simulink model "rx2"  (R2022b)
settings: Solver=FixedStepDiscrete  StartTime=0.0  StopTime=3.3E6  FixedStep=1  RelTol=1e-3  EnableMultiTasking=on
model workspace (MAT data in the model file):
  mwTaskManagerKernelLatency = 0
undefined symbols (not defined in the file or in its folder): Add, jsin, magnitude, rom_pilot_conj_tt, Shift
libraries: hdlsllib x3231, whdlutilities x525, simulink x260, whdlmod x112, whdledac x26, dsphdlmathfun2 x24, commchan3 x1
(part 8 of 59)

== system rx2/process11/decoder/p-p ==
  data_in : Inport  OutDataTypeStr=boolean  PortDimensions=64
  start_in : Inport  Port=2  OutDataTypeStr=boolean  PortDimensions=1
  valid : Inport  Port=3  OutDataTypeStr=boolean  PortDimensions=1
  Compare To Constant : hdlsllib/Logic and Bit Operations/Compare To Constant  relop===  const=64  OutDataTypeStr=boolean
  Compare To Constant1 : hdlsllib/Logic and Bit Operations/Compare To Constant  relop=<=  const=72  OutDataTypeStr=boolean
  Compare To Constant2 : hdlsllib/Logic and Bit Operations/Compare To Constant  relop===  const=1  OutDataTypeStr=boolean
  Compare To Constant3 : hdlsllib/Logic and Bit Operations/Compare To Constant  relop===  const=528  OutDataTypeStr=boolean
  Compare To Constant4 : hdlsllib/Logic and Bit Operations/Compare To Constant  relop=<=  const=528  OutDataTypeStr=boolean
  Delay : Delay  DelayLength=1  InitialCondition=0
  Delay1 : Delay  DelayLength=1  InitialCondition=0
  Ground : Ground
  HDL Counter : hdlsllib/Sources/HDL Counter  CountType=Count limited  CountInit=0  CountStep=1  CountMax=2000  CountFromType=Specify  CountFrom=0  CountResetPort=on  CountLoadPort=off  CountEnbPort=on  CountDirPort=off  CountHitOutputPort=off  CountDataType=Unsigned  CountWordLen=16  CountFracLen=0  CountSampTime=1
  HDL Counter1 : hdlsllib/Sources/HDL Counter  CountType=Count limited  CountInit=1  CountStep=1  CountMax=64  CountFromType=Specify  CountFrom=1  CountResetPort=on  CountLoadPort=off  CountEnbPort=on  CountDirPort=off  CountHitOutputPort=off  CountDataType=Unsigned  CountWordLen=16  CountFracLen=0  CountSampTime=1
  HDL Counter2 : hdlsllib/Sources/HDL Counter  CountType=Count limited  CountInit=0  CountStep=1  CountMax=100  CountFromType=Specify  CountFrom=0  CountResetPort=on  CountLoadPort=off  CountEnbPort=on  CountDirPort=off  CountHitOutputPort=off  CountDataType=Unsigned  CountWordLen=16  CountFracLen=0  CountSampTime=1
  HDL Counter3 : hdlsllib/Sources/HDL Counter  CountType=Count limited  CountInit=1  CountStep=1  CountMax=64*2  CountFromType=Initial value  CountFrom=1  CountResetPort=on  CountLoadPort=off  CountEnbPort=on  CountDirPort=off  CountHitOutputPort=off  CountDataType=Unsigned  CountWordLen=8  CountFracLen=0  CountSampTime=1
  HDL Counter4 : hdlsllib/Sources/HDL Counter  CountType=Count limited  CountInit=0  CountStep=1  CountMax=1000  CountFromType=Initial value  CountFrom=0  CountResetPort=on  CountLoadPort=off  CountEnbPort=on  CountDirPort=off  CountHitOutputPort=off  CountDataType=Unsigned  CountWordLen=16  CountFracLen=0  CountSampTime=1
  HDL Counter5 : hdlsllib/Sources/HDL Counter  CountType=Count limited  CountInit=1  CountStep=1  CountMax=1000  CountFromType=Initial value  CountFrom=1  CountResetPort=on  CountLoadPort=off  CountEnbPort=on  CountDirPort=off  CountHitOutputPort=off  CountDataType=Unsigned  CountWordLen=16  CountFracLen=0  CountSampTime=1
  Logical Operator1 : Logic  Operator=NOT  AllPortsSameDT=off  OutDataTypeStr=boolean
  Logical Operator2 : Logic  Operator=NOT  AllPortsSameDT=off  OutDataTypeStr=boolean
  Logical Operator3 : Logic  AllPortsSameDT=off  OutDataTypeStr=boolean
  Logical Operator5 : Logic  Operator=NOT  AllPortsSameDT=off  OutDataTypeStr=boolean
  Logical Operator6 : Logic  AllPortsSameDT=off  OutDataTypeStr=boolean
  Sample Control Bus Creator : whdlutilities/Sample Control Bus Creator
  Subsystem : Subsystem  mask{valid_length=20*64}
      mask prompts: valid_length "The length of valid"
      mask DialogControl Control2 Prompt: Latency=2
  Subsystem2 : Subsystem  mask{data_type=boolean, address_len=16}
      mask prompts: data_type "the type of input data"; address_len "the length of address"
      mask DialogControl ParameterGroupVar Prompt: 参数
  Switch : Switch  Criteria=u2 ~= 0  SaturateOnIntegerOverflow=off  InputSameDT=off
  p_s_new : Subsystem
  data : Outport
  ctrl : Outport  Port=2
  wires:
  Ground/1 -> Switch/3
  Switch/1 -> data/1
  Subsystem/3(end_out) -> p_s_new/3(end)
  p_s_new/1(data_out) -> Delay1/1
  Subsystem2/1(rd_dout) -> p_s_new/1(data_in)
  Subsystem/1(valid_out) -> HDL Counter1/2, Logical Operator1/1, HDL Counter3/2, Logical Operator2/1, Logical Operator3/1, p_s_new/2(valid)
  Logical Operator6/1 -> HDL Counter4/2, Delay/1
  Compare To Constant4/1 -> Logical Operator6/1
  HDL Counter5/1 -> Compare To Constant4/1
  Sample Control Bus Creator/1 -> ctrl/1
  Delay1/1 -> Switch/1
  Delay/1 -> Sample Control Bus Creator/3, Switch/2
  Compare To Constant3/1 -> HDL Counter4/1, Sample Control Bus Creator/2
  Compare To Constant2/1 -> Sample Control Bus Creator/1
  HDL Counter1/1 -> Compare To Constant/1
  Compare To Constant1/1 -> Logical Operator3/2
  HDL Counter3/1 -> Compare To Constant1/1
  HDL Counter2/1 -> Subsystem2/4(rd_addr)
  data_in/1 -> Subsystem2/1(data1)
  Logical Operator5/1 -> HDL Counter/1
  Logical Operator2/1 -> HDL Counter3/1, HDL Counter5/1
  Compare To Constant/1 -> HDL Counter2/2
  start_in/1 -> Subsystem/1(start)
  HDL Counter/1 -> Subsystem2/2(wr_addr)
  valid/1 -> Logical Operator5/1, Subsystem2/3(wr_en1), HDL Counter/2
  Logical Operator3/1 -> Logical Operator6/2, HDL Counter5/2
  Logical Operator1/1 -> HDL Counter1/1, HDL Counter2/1
  HDL Counter4/1 -> Compare To Constant2/1, Compare To Constant3/1

== system rx2/process11/decoder/rate recover ==
  demod : Inport
  valid_in : Inport  Port=2
  start_in : Inport  Port=3
  Compare To Constant : hdlsllib/Logic and Bit Operations/Compare To Constant  relop=<=  const=384  OutDataTypeStr=boolean
  Compare To Constant1 : hdlsllib/Logic and Bit Operations/Compare To Constant  relop=>=  const=577  OutDataTypeStr=boolean
  Compare To Constant2 : hdlsllib/Logic and Bit Operations/Compare To Constant  relop=<=  const=1776  OutDataTypeStr=boolean
  Compare To Constant3 : hdlsllib/Logic and Bit Operations/Compare To Constant  relop=>=  const=385  OutDataTypeStr=boolean
  Compare To Constant4 : hdlsllib/Logic and Bit Operations/Compare To Constant  relop=<=  const=576  OutDataTypeStr=boolean
  Compare To Constant5 : hdlsllib/Logic and Bit Operations/Compare To Constant  relop=>=  const=1777  OutDataTypeStr=boolean
  Compare To Constant6 : hdlsllib/Logic and Bit Operations/Compare To Constant  relop=<=  const=3600  OutDataTypeStr=boolean
  Constant : Constant  Value=0
  Constant1 : Constant  Value=0
  Delay{,1..4} (5 alike) : Delay  InitialCondition=0
  HDL Counter : hdlsllib/Sources/HDL Counter  CountType=Count limited  CountInit=1  CountStep=1  CountMax=10000  CountFromType=Initial value  CountFrom=1  CountResetPort=on  CountLoadPort=off  CountEnbPort=on  CountDirPort=off  CountHitOutputPort=off  CountDataType=Unsigned  CountWordLen=16  CountFracLen=0  CountSampTime=1
  HDL Counter1 : hdlsllib/Sources/HDL Counter  CountType=Count limited  CountInit=0  CountStep=1  CountMax=10000  CountFromType=Initial value  CountFrom=0  CountResetPort=on  CountLoadPort=off  CountEnbPort=on  CountDirPort=off  CountHitOutputPort=off  CountDataType=Unsigned  CountWordLen=16  CountFracLen=0  CountSampTime=1
  HDL Counter3 : hdlsllib/Sources/HDL Counter  CountType=Count limited  CountInit=1  CountStep=1  CountMax=10000  CountFromType=Initial value  CountFrom=1  CountResetPort=on  CountLoadPort=off  CountEnbPort=on  CountDirPort=off  CountHitOutputPort=off  CountDataType=Unsigned  CountWordLen=16  CountFracLen=0  CountSampTime=1
  Logical Operator : Logic  Operator=NOT  AllPortsSameDT=off  OutDataTypeStr=boolean
  Logical Operator{1,3..4,6..7} (5 alike) : Logic  AllPortsSameDT=off  OutDataTypeStr=boolean
  Logical Operator5 : Logic  Operator=OR  AllPortsSameDT=off  OutDataTypeStr=boolean
  Logical Operator8 : Logic  Operator=NOT  AllPortsSameDT=off  OutDataTypeStr=boolean
  Simple Dual Port RAM : hdlsllib/HDL RAMs/Simple Dual Port RAM  ram_size=16
  Subsystem : Subsystem  mask{valid_length=3600}
      mask prompts: valid_length "The length of valid"
      mask DialogControl Control2 Prompt: Latency=2
  Switch : Switch  Criteria=u2 ~= 0  SaturateOnIntegerOverflow=off  InputSameDT=off
  Switch1 : Switch  Criteria=u2 ~= 0  OutDataTypeStr=fixdt(1,16,9)  SaturateOnIntegerOverflow=off  InputSameDT=off
  rate_recover : Outport  PortDimensions=1
  start_out : Outport  Port=2  OutDataTypeStr=boolean
  end_out : Outport  Port=3  OutDataTypeStr=boolean
  valid_out : Outport  Port=4  OutDataTypeStr=boolean
  wires:
  Compare To Constant5/1 -> Logical Operator4/1
  Logical Operator3/1 -> Delay3/1
  Subsystem/1(valid_out) -> Logical Operator8/1, Logical Operator6/2, Delay/1, HDL Counter3/2
  Constant1/1 -> Switch1/1
  Subsystem/2(start_out) -> Delay1/1  "start"
  Logical Operator/1 -> HDL Counter/1
  Logical Operator1/1 -> Logical Operator5/2
  Compare To Constant3/1 -> Logical Operator3/1
  Subsystem/3(end_out) -> Delay2/1  "end"
  HDL Counter/1 -> Simple Dual Port RAM/2  "wr_addr"
  Compare To Constant6/1 -> Logical Operator4/2
  Compare To Constant1/1 -> Logical Operator1/1
  Compare To Constant2/1 -> Logical Operator1/2
  valid_in/1 -> Simple Dual Port RAM/3, HDL Counter/2, Logical Operator/1
  Delay1/1 -> start_out/1  "start_out"
  Logical Operator7/1 -> Delay4/1  "3"
  Simple Dual Port RAM/1 -> Switch/3  "rd_dout"
  start_in/1 -> Subsystem/1(start)
  Compare To Constant4/1 -> Logical Operator3/2
  Logical Operator4/1 -> Logical Operator7/1
  Constant/1 -> Switch/1
  Switch/1 -> Switch1/3  "2_out"
  Switch1/1 -> rate_recover/1  "data_out"
  Logical Operator5/1 -> Logical Operator6/1
  Compare To Constant/1 -> Logical Operator5/1
  Delay2/1 -> end_out/1  "end_out"
  demod/1 -> Simple Dual Port RAM/1
  Delay/1 -> Logical Operator7/2, valid_out/1  "valid_out"
  Logical Operator8/1 -> HDL Counter1/1, HDL Counter3/1
  HDL Counter3/1 -> Compare To Constant1/1, Compare To Constant/1, Compare To Constant6/1, Compare To Constant5/1, Compare To Constant4/1, Compare To Constant3/1, Compare To Constant2/1  "count"
  Delay3/1 -> Switch/2  "2"
  Delay4/1 -> Switch1/2  "3"
  Logical Operator6/1 -> HDL Counter1/2  "1"
  HDL Counter1/1 -> Simple Dual Port RAM/4  "rd_addr"

== system rx2/process11/decoder/s-p ==
  data_in : Inport
  valid_in : Inport  Port=2
  Compare To Constant1 : hdlsllib/Logic and Bit Operations/Compare To Constant  relop=<=  const=64  OutDataTypeStr=boolean
  Compare To Constant2 : hdlsllib/Logic and Bit Operations/Compare To Constant  relop===  const=2  OutDataTypeStr=boolean
  Compare To Constant3 : hdlsllib/Logic and Bit Operations/Compare To Constant  relop===  const=3  OutDataTypeStr=boolean
  Compare To Constant4 : hdlsllib/Logic and Bit Operations/Compare To Constant  relop===  const=1  OutDataTypeStr=boolean
  Compare To Constant5 : hdlsllib/Logic and Bit Operations/Compare To Constant  relop===  const=100  OutDataTypeStr=boolean
  Constant2 : Constant  Value=2  OutDataTypeStr=uint8
  Constant3 : Constant  Value=zeros(1,56)  OutDataTypeStr=fixdt(1,16,9)
  Delay1 : Delay  DelayLength=1  InitialCondition=0
  Delay4 : Delay  DelayLength=1  InitialCondition=0
  HDL Counter : hdlsllib/Sources/HDL Counter  CountType=Count limited  CountInit=1  CountStep=1  CountMax=72  CountFromType=Initial value  CountFrom=1  CountResetPort=on  CountLoadPort=off  CountEnbPort=on  CountDirPort=off  CountHitOutputPort=off  CountDataType=Unsigned  CountWordLen=8  CountFracLen=0  CountSampTime=1
  HDL Counter1 : hdlsllib/Sources/HDL Counter  CountType=Count limited  CountInit=1  CountStep=1  CountMax=72  CountFromType=Initial value  CountFrom=1  CountResetPort=on  CountLoadPort=off  CountEnbPort=on  CountDirPort=off  CountHitOutputPort=off  CountDataType=Unsigned  CountWordLen=8  CountFracLen=0  CountSampTime=1
  HDL Counter2 : hdlsllib/Sources/HDL Counter  CountType=Count limited  CountInit=1  CountStep=1  CountMax=72  CountFromType=Initial value  CountFrom=1  CountResetPort=on  CountLoadPort=off  CountEnbPort=on  CountDirPort=off  CountHitOutputPort=off  CountDataType=Unsigned  CountWordLen=8  CountFracLen=0  CountSampTime=1
  HDL Counter3 : hdlsllib/Sources/HDL Counter  CountType=Count limited  CountInit=0  CountStep=1  CountMax=200  CountFromType=Initial value  CountFrom=0  CountResetPort=on  CountLoadPort=off  CountEnbPort=on  CountDirPort=off  CountHitOutputPort=off  CountDataType=Unsigned  CountWordLen=8  CountFracLen=0  CountSampTime=1
  Logical Operator{1,5..6,8} (4 alike) : Logic  Operator=NOT  AllPortsSameDT=off  OutDataTypeStr=boolean
  Logical Operator2 : Logic  Operator=XOR  AllPortsSameDT=off  OutDataTypeStr=boolean
  Logical Operator3 : Logic  AllPortsSameDT=off  OutDataTypeStr=boolean
  Logical Operator4 : Logic  AllPortsSameDT=off  OutDataTypeStr=boolean
  Mod : Math  Operator=mod
  Mux : Mux  Inputs=2
  S-P : Subsystem  mask{data_len=64}
      mask prompts: data_len "the length of parallel"
      mask DialogControl ParameterGroupVar Prompt: 参数
  S-P2 : Subsystem  mask{data_len=8}
      mask prompts: data_len "the length of parallel"
      mask DialogControl ParameterGroupVar Prompt: 参数
  Sample Control Bus Creator : whdlutilities/Sample Control Bus Creator
  Switch1 : Switch  Criteria=u2 ~= 0  OutDataTypeStr=Inherit: Inherit via back propagation  SaturateOnIntegerOverflow=off  InputSameDT=off
  data_out : Outport
  ctrl_out : Outport  Port=2
  wires:
  Compare To Constant1/1 -> Logical Operator8/1, Logical Operator3/2
  Logical Operator2/1 -> Delay1/1, HDL Counter3/2  "valid"
  Logical Operator4/1 -> Sample Control Bus Creator/1  "start"
  HDL Counter/1 -> Compare To Constant1/1
  Compare To Constant2/1 -> Logical Operator2/1, Delay4/1
  S-P2/2(valid_out) -> HDL Counter2/2, Logical Operator6/1
  HDL Counter1/1 -> Compare To Constant2/1
  data_in/1 -> S-P2/1(data_in), S-P/1(data_in)
  valid_in/1 -> Logical Operator1/1, Logical Operator3/1, HDL Counter/2
  Sample Control Bus Creator/1 -> ctrl_out/1
  Constant3/1 -> Mux/2
  HDL Counter3/1 -> Mod/1, Compare To Constant4/1, Compare To Constant5/1
  Compare To Constant3/1 -> Logical Operator2/2
  Mod/1 -> Switch1/2
  Switch1/1 -> data_out/1
  Constant2/1 -> Mod/2
  S-P2/1(data_out) -> Mux/1
  Mux/1 -> Switch1/3
  HDL Counter2/1 -> Compare To Constant3/1
  Logical Operator8/1 -> S-P2/2(valid_in)
  S-P/2(valid_out) -> HDL Counter1/2, Logical Operator5/1  "validout"
  S-P/1(data_out) -> Switch1/1
  Logical Operator3/1 -> S-P/2(valid_in)
  Logical Operator1/1 -> HDL Counter/1
  Logical Operator5/1 -> HDL Counter1/1
  Logical Operator6/1 -> HDL Counter2/1
  Compare To Constant5/1 -> Sample Control Bus Creator/2, HDL Counter3/1  "start"
  Compare To Constant4/1 -> Logical Operator4/2
  Delay4/1 -> Logical Operator4/1
  Delay1/1 -> Sample Control Bus Creator/3

== system rx2/process11/decoder/soft demodule ==
  nVar_tt : Inport  OutDataTypeStr=fixdt(0,16,12)
  G_k_1 : Inport  Port=2
  r_k : Inport  Port=3
  start : Inport  Port=4
  valid : Inport  Port=5
  Complex to Real-Imag : ComplexToRealImag
  Constant1 : Constant  Value=2  OutDataTypeStr=uint16
  Constant2 : Constant  Value=2  OutDataTypeStr=uint16
  Constant3 : Constant  Value=0  OutDataTypeStr=uint16
  Constant4 : Constant  Value=0  OutDataTypeStr=uint16
  Data Type Conversion2 : DataTypeConversion  OutDataTypeStr=boolean  SaturateOnIntegerOverflow=off  RndMeth=Floor
  Delay1 : Delay  InitialCondition=0
  Delay2 : Delay  DelayLength=1  InitialCondition=0
  Delay3 : Delay  InitialCondition=0
  Delay4 : Delay  InitialCondition=0
  HDL Counter : hdlsllib/Sources/HDL Counter  CountType=Count limited  CountInit=1  CountStep=1  CountMax=2000  CountFromType=Initial value  CountFrom=1  CountResetPort=on  CountLoadPort=off  CountEnbPort=on  CountDirPort=off  CountHitOutputPort=off  CountDataType=Unsigned  CountWordLen=16  CountFracLen=0  CountSampTime=1
  HDL Counter2 : hdlsllib/Sources/HDL Counter  CountType=Count limited  CountInit=1  CountStep=1  CountMax=2000  CountFromType=Initial value  CountFrom=1  CountResetPort=on  CountLoadPort=off  CountEnbPort=on  CountDirPort=off  CountHitOutputPort=off  CountDataType=Unsigned  CountWordLen=16  CountFracLen=0  CountSampTime=1
  HDL Counter3 : hdlsllib/Sources/HDL Counter  CountType=Count limited  CountInit=0  CountStep=1  CountMax=2000  CountFromType=Initial value  CountFrom=0  CountResetPort=on  CountLoadPort=off  CountEnbPort=on  CountDirPort=off  CountHitOutputPort=off  CountDataType=Unsigned  CountWordLen=16  CountFracLen=0  CountSampTime=1
  HDL Counter5 : hdlsllib/Sources/HDL Counter  CountType=Count limited  CountInit=0  CountStep=1  CountMax=2000  CountFromType=Initial value  CountFrom=0  CountResetPort=on  CountLoadPort=off  CountEnbPort=on  CountDirPort=off  CountHitOutputPort=off  CountDataType=Unsigned  CountWordLen=16  CountFracLen=0  CountSampTime=1
  Logical Operator2 : Logic  AllPortsSameDT=off  OutDataTypeStr=boolean
  Logical Operator3 : Logic  Operator=NOT  AllPortsSameDT=off  OutDataTypeStr=boolean
  Logical Operator4 : Logic  Operator=NOT  AllPortsSameDT=off  OutDataTypeStr=boolean
  Logical Operator5 : Logic  Operator=NOT  AllPortsSameDT=off  OutDataTypeStr=boolean
  Logical Operator6 : Logic  Operator=XOR  AllPortsSameDT=off  OutDataTypeStr=boolean
  Math Reciprocal2 : Math  Operator=reciprocal  SignedPower=on  OutDataTypeStr=fixdt(1,16,12)
  Mod : Math  Operator=mod  SignedPower=on
  Product : Product
  Product1 : Product
  Product10 : Product  OutDataTypeStr=fixdt(1,35,24)
  Product2 : Product  OutDataTypeStr=fixdt(1,35,24)
  Simple Dual Port RAM : hdlsllib/HDL RAMs/Simple Dual Port RAM  ram_size=16
  Simple Dual Port RAM1 : hdlsllib/HDL RAMs/Simple Dual Port RAM  ram_size=16
  Subsystem : Subsystem  mask{valid_length=demod_length}
      mask prompts: valid_length "The length of valid"
      mask DialogControl Control2 Prompt: Latency=2
  Switch : Switch  Criteria=u2 ~= 0  SaturateOnIntegerOverflow=off  InputSameDT=off
  Switch1 : Switch  Criteria=u2 ~= 0  SaturateOnIntegerOverflow=off  InputSameDT=off
  Switch2 : Switch  Criteria=u2 ~= 0  SaturateOnIntegerOverflow=off  InputSameDT=off
  demod : Outport  OutDataTypeStr=fixdt(1,16,9)  VectorParamsAs1DForOutWhenUnconnected=off
  valid_out : Outport  Port=2  OutDataTypeStr=boolean  VectorParamsAs1DForOutWhenUnconnected=off
  start_out : Outport  Port=3  OutDataTypeStr=boolean  VectorParamsAs1DForOutWhenUnconnected=off
  end_out : Outport  Port=4  OutDataTypeStr=boolean  VectorParamsAs1DForOutWhenUnconnected=off
  wires:
  valid/1 -> Switch2/2, Switch1/2, Simple Dual Port RAM1/3, Simple Dual Port RAM/3, HDL Counter2/2, Logical Operator4/1  "valid_tt"
  start/1 -> Subsystem/1(start)
  Logical Operator2/1 -> Logical Operator6/2, HDL Counter3/2  "mod_1"
  Complex to Real-Imag/2 -> Product1/2  "r_k_imag"
  Subsystem/1(valid_out) -> Delay1/1, HDL Counter/2, Logical Operator3/1, Logical Operator2/2, Logical Operator6/1, Logical Operator5/1
  Product/1 -> Switch1/1  "demod_1"
  Product1/1 -> Switch2/1  "demod_0"
  Switch/1 -> demod/1  "demod"
  Mod/1 -> Data Type Conversion2/1  "mod"
  Logical Operator6/1 -> Delay2/1, HDL Counter5/2  "mod_0"
  Complex to Real-Imag/1 -> Product/2  "r_k_real"
  Logical Operator4/1 -> HDL Counter2/1
  HDL Counter3/1 -> Simple Dual Port RAM/4  "rd_addr1"
  Logical Operator5/1 -> HDL Counter5/1, HDL Counter3/1  "rst"
  Logical Operator3/1 -> HDL Counter/1
  Constant1/1 -> Mod/2
  HDL Counter5/1 -> Simple Dual Port RAM1/4  "rd_addr0"
  Simple Dual Port RAM/1 -> Switch/1  "demod_11"
  HDL Counter2/1 -> Simple Dual Port RAM1/2, Simple Dual Port RAM/2  "wr_addr"
  Simple Dual Port RAM1/1 -> Switch/3  "demod_00"
  Data Type Conversion2/1 -> Logical Operator2/1
  Delay1/1 -> valid_out/1  "valid_out"
  HDL Counter/1 -> Mod/1  "count"
  nVar_tt/1 -> Math Reciprocal2/1  "nvar"
  G_k_1/1 -> Product10/2  "G_k_1"
  r_k/1 -> Complex to Real-Imag/1  "r_k"
  Subsystem/2(start_out) -> Delay3/1
  Subsystem/3(end_out) -> Delay4/1
  Delay2/1 -> Switch/2
  Delay3/1 -> start_out/1  "start_out"
  Delay4/1 -> end_out/1  "end_out"
  Math Reciprocal2/1 -> Product10/1  "nvar"
  Product10/1 -> Product2/2
  Product2/1 -> Product1/1, Product/1
  Constant2/1 -> Product2/1
  Constant3/1 -> Switch1/3
  Switch1/1 -> Simple Dual Port RAM/1  "demod1"
  Constant4/1 -> Switch2/3
  Switch2/1 -> Simple Dual Port RAM1/1  "demod0"

== system rx2/process11/decoder/synchronization ==
  chan_est_tt : Inport
  rxSig_tt : Inport  Port=2
  port1_ctrl : Inport  Port=3  OutDataTypeStr=Bus: BUSOFDM1
  port2_ctrl : Inport  Port=4  OutDataTypeStr=Bus: BUSOFDM1
  Bus Selector1 : BusSelector  OutputSignals=signal1,signal2,signal3,signal4,signal5,signal6,signal7,signal8
  Bus Selector2 : BusSelector  OutputSignals=OFDM_ctrl_bf1_process1,OFDM_ctrl_bf1_process2,OFDM_ctrl_bf1_process3,OFDM_ctrl_bf1_process4,OFDM_ctrl_bf1_process5,OFDM_ctrl_bf1_process6,OFDM_ctrl_bf1_process7,OFDM_ctrl_bf1_process8
  Demux : Demux  Outputs=8
  Demux1 : Demux  Outputs=8
  Mux : Mux  Inputs=8
  Mux1 : Mux  Inputs=8
  data_synchronization1 : Subsystem
  data_synchronization2 : Subsystem
  data_synchronization3 : Subsystem
  data_synchronization4 : Subsystem
  data_synchronization5 : Subsystem
  data_synchronization6 : Subsystem
  data_synchronization7 : Subsystem
  data_synchronization8 : Subsystem
  port1_syn : Outport
  port2_syn : Outport  Port=2
  valid_syn : Outport  Port=3
  wires:
  Bus Selector2/3 -> data_synchronization8/4(port2_ctrl)  "<OFDM_ctrl_bf1_process3>"
  Bus Selector2/4 -> data_synchronization7/4(port2_ctrl)  "<OFDM_ctrl_bf1_process4>"
  Bus Selector2/5 -> data_synchronization6/4(port2_ctrl)  "<OFDM_ctrl_bf1_process5>"
  Bus Selector2/6 -> data_synchronization5/4(port2_ctrl)  "<OFDM_ctrl_bf1_process6>"
  Bus Selector2/7 -> data_synchronization4/4(port2_ctrl)  "<OFDM_ctrl_bf1_process7>"
  Bus Selector2/8 -> data_synchronization3/4(port2_ctrl)  "<OFDM_ctrl_bf1_process8>"
  Bus Selector2/2 -> data_synchronization2/4(port2_ctrl)  "<OFDM_ctrl_bf1_process2>"
  Bus Selector2/1 -> data_synchronization1/4(port2_ctrl)  "<OFDM_ctrl_bf1_process1>"
  port2_ctrl/1 -> Bus Selector2/1
  Bus Selector1/8 -> data_synchronization8/3(port1_ctrl)  "<signal8>"
  Bus Selector1/7 -> data_synchronization7/3(port1_ctrl)  "<signal7>"
  Bus Selector1/6 -> data_synchronization6/3(port1_ctrl)  "<signal6>"
  Bus Selector1/5 -> data_synchronization5/3(port1_ctrl)  "<signal5>"
  Bus Selector1/4 -> data_synchronization4/3(port1_ctrl)  "<signal4>"
  Bus Selector1/3 -> data_synchronization3/3(port1_ctrl)  "<signal3>"
  Bus Selector1/2 -> data_synchronization2/3(port1_ctrl)  "<signal2>"
  Bus Selector1/1 -> data_synchronization1/3(port1_ctrl)  "<signal1>"
  port1_ctrl/1 -> Bus Selector1/1
  rxSig_tt/1 -> Demux1/1
  data_synchronization6/3(valid_syn) -> ?
  chan_est_tt/1 -> Demux/1
  data_synchronization4/4(start_syn) -> ?
  data_synchronization2/3(valid_syn) -> ?
  data_synchronization4/3(valid_syn) -> ?
  data_synchronization6/4(start_syn) -> ?
  data_synchronization7/3(valid_syn) -> ?
  data_synchronization3/3(valid_syn) -> ?
  data_synchronization5/3(valid_syn) -> ?
  data_synchronization8/4(start_syn) -> ?
  Demux1/5 -> data_synchronization5/2(port2)
  Demux1/3 -> data_synchronization3/2(port2)
  data_synchronization2/4(start_syn) -> ?
  data_synchronization3/2(port2_syn) -> Mux1/3
  data_synchronization7/1(port1_syn) -> Mux/7
  Demux1/1 -> data_synchronization1/2(port2)
  Demux/8 -> data_synchronization8/1(port1)
  data_synchronization1/1(port1_syn) -> Mux/1
  Demux/3 -> data_synchronization3/1(port1)
  data_synchronization3/4(start_syn) -> ?
  data_synchronization1/3(valid_syn) -> valid_syn/1
  data_synchronization1/2(port2_syn) -> Mux1/1
  Demux/4 -> data_synchronization4/1(port1)
  data_synchronization5/4(start_syn) -> ?
  data_synchronization8/1(port1_syn) -> Mux/8
  Demux/6 -> data_synchronization6/1(port1)
  data_synchronization7/2(port2_syn) -> Mux1/7
  data_synchronization6/1(port1_syn) -> Mux/6
  Demux/7 -> data_synchronization7/1(port1)
  Demux/1 -> data_synchronization1/1(port1)
  data_synchronization4/2(port2_syn) -> Mux1/4
  data_synchronization4/1(port1_syn) -> Mux/4
  data_synchronization5/2(port2_syn) -> Mux1/5
  data_synchronization5/1(port1_syn) -> Mux/5
  Mux1/1 -> port2_syn/1
  Demux1/4 -> data_synchronization4/2(port2)
  Demux1/6 -> data_synchronization6/2(port2)
  data_synchronization8/2(port2_syn) -> Mux1/8
  data_synchronization2/2(port2_syn) -> Mux1/2
  data_synchronization7/4(start_syn) -> ?
  data_synchronization6/2(port2_syn) -> Mux1/6
  Demux/5 -> data_synchronization5/1(port1)
  Demux1/8 -> data_synchronization8/2(port2)
  data_synchronization8/3(valid_syn) -> ?
  Demux1/7 -> data_synchronization7/2(port2)
  data_synchronization2/1(port1_syn) -> Mux/2
  Mux/1 -> port1_syn/1
  Demux1/2 -> data_synchronization2/2(port2)
  Demux/2 -> data_synchronization2/1(port1)
  data_synchronization3/1(port1_syn) -> Mux/3

== system rx2/process11/decoder/synchronize_valid ==
  start : Inport
  Compare To Constant : simulink/Logic and Bit Operations/Compare To Constant  relop===  const=valid_length  OutDataTypeStr=boolean
  Data Type Conversion : DataTypeConversion  OutDataTypeStr=boolean  SaturateOnIntegerOverflow=off  RndMeth=Floor
  Delay2 : Delay  DelayLength=1  InitialCondition=0
  HDL Counter1 : hdlsllib/Sources/HDL Counter  CountType=Count limited  CountInit=1  CountStep=1  CountMax=valid_length  CountFromType=Initial value  CountFrom=1  CountResetPort=off  CountLoadPort=off  CountEnbPort=on  CountDirPort=off  CountHitOutputPort=off  CountDataType=Unsigned  CountWordLen=16  CountFracLen=0  CountSampTime=1
  HDL Counter4 : hdlsllib/Sources/HDL Counter  CountType=Count limited  CountInit=0  CountStep=1  CountMax=1  CountFromType=Initial value  CountFrom=0  CountResetPort=on  CountLoadPort=off  CountEnbPort=on  CountDirPort=off  CountHitOutputPort=off  CountDataType=Unsigned  CountWordLen=8  CountFracLen=0  CountSampTime=1
  valid_out : Outport
  wires:
  Compare To Constant/1 -> HDL Counter4/1
  HDL Counter1/1 -> Compare To Constant/1  "count_1"
  HDL Counter4/1 -> Data Type Conversion/1
  start/1 -> HDL Counter4/2
  Data Type Conversion/1 -> Delay2/1, HDL Counter1/1
  Delay2/1 -> valid_out/1  "valid_out"

== system rx2/process12/OFDM_DEMOD1/OFDM_demod1 ==
  ofdm_sym : Inport
  valid_in : Inport  Port=2  OutDataTypeStr=boolean
  OFDM Demodulator : whdlmod/OFDM Demodulator  OFDMParamsSource=Property  MaxFFTLength=64  FFTLength=1024  CPLength=72  NumLGsC=0  NumRGsC=0  CPFraction=off  CPFractionValue=0.55  removeDCSubcarriers=off  enableResetInputPort=off  Normalize=off  RoundingMethod=Floor  SimulateUsing=Code generation
  ctrl_gen : Subsystem
  data_out : Outport  OutDataTypeStr=fixdt(1,16,12)
  ctrl_out : Outport  Port=2  OutDataTypeStr=Bus: samplecontrol
  wires:
  ofdm_sym/1 -> OFDM Demodulator/1
  valid_in/1 -> OFDM Demodulator/2
  OFDM Demodulator/1 -> ctrl_gen/1(data_in)
  ctrl_gen/1(data_out) -> data_out/1
  OFDM Demodulator/2 -> ctrl_gen/2(valid_in)
  ctrl_gen/2(ctrl_out) -> ctrl_out/1

== system rx2/process12/OFDM_DEMOD1/OFDM_demod2 ==
  ofdm_sym : Inport
  valid_in : Inport  Port=2  OutDataTypeStr=boolean
  OFDM Demodulator : whdlmod/OFDM Demodulator  OFDMParamsSource=Property  MaxFFTLength=64  FFTLength=1024  CPLength=72  NumLGsC=0  NumRGsC=0  CPFraction=off  CPFractionValue=0.55  removeDCSubcarriers=off  enableResetInputPort=off  Normalize=off  RoundingMethod=Floor  SimulateUsing=Code generation
  ctrl_gen : Subsystem
  data_out : Outport  OutDataTypeStr=fixdt(1,16,12)
  ctrl_out : Outport  Port=2  OutDataTypeStr=Bus: samplecontrol
  wires:
  ofdm_sym/1 -> OFDM Demodulator/1
  valid_in/1 -> OFDM Demodulator/2
  OFDM Demodulator/1 -> ctrl_gen/1(data_in)
  ctrl_gen/1(data_out) -> data_out/1
  OFDM Demodulator/2 -> ctrl_gen/2(valid_in)
  ctrl_gen/2(ctrl_out) -> ctrl_out/1

== system rx2/process12/OFDM_DEMOD1/OFDM_demod3 ==
  ofdm_sym : Inport
  valid_in : Inport  Port=2  OutDataTypeStr=boolean
  OFDM Demodulator : whdlmod/OFDM Demodulator  OFDMParamsSource=Property  MaxFFTLength=64  FFTLength=1024  CPLength=72  NumLGsC=0  NumRGsC=0  CPFraction=off  CPFractionValue=0.55  removeDCSubcarriers=off  enableResetInputPort=off  Normalize=off  RoundingMethod=Floor  SimulateUsing=Code generation
  ctrl_gen : Subsystem
  data_out : Outport  OutDataTypeStr=fixdt(1,16,12)
  ctrl_out : Outport  Port=2  OutDataTypeStr=Bus: samplecontrol
  wires:
  ofdm_sym/1 -> OFDM Demodulator/1
  valid_in/1 -> OFDM Demodulator/2
  OFDM Demodulator/1 -> ctrl_gen/1(data_in)
  ctrl_gen/1(data_out) -> data_out/1
  OFDM Demodulator/2 -> ctrl_gen/2(valid_in)
  ctrl_gen/2(ctrl_out) -> ctrl_out/1

== system rx2/process12/OFDM_DEMOD1/OFDM_demod4 ==
  ofdm_sym : Inport
  valid_in : Inport  Port=2  OutDataTypeStr=boolean
  OFDM Demodulator : whdlmod/OFDM Demodulator  OFDMParamsSource=Property  MaxFFTLength=64  FFTLength=1024  CPLength=72  NumLGsC=0  NumRGsC=0  CPFraction=off  CPFractionValue=0.55  removeDCSubcarriers=off  enableResetInputPort=off  Normalize=off  RoundingMethod=Floor  SimulateUsing=Code generation
  ctrl_gen : Subsystem
  data_out : Outport  OutDataTypeStr=fixdt(1,16,12)
  ctrl_out : Outport  Port=2  OutDataTypeStr=Bus: samplecontrol
  wires:
  ofdm_sym/1 -> OFDM Demodulator/1
  valid_in/1 -> OFDM Demodulator/2
  OFDM Demodulator/1 -> ctrl_gen/1(data_in)
  ctrl_gen/1(data_out) -> data_out/1
  OFDM Demodulator/2 -> ctrl_gen/2(valid_in)
  ctrl_gen/2(ctrl_out) -> ctrl_out/1

== system rx2/process12/OFDM_DEMOD1/OFDM_demod5 ==
  ofdm_sym : Inport
  valid_in : Inport  Port=2  OutDataTypeStr=boolean
  OFDM Demodulator : whdlmod/OFDM Demodulator  OFDMParamsSource=Property  MaxFFTLength=64  FFTLength=1024  CPLength=72  NumLGsC=0  NumRGsC=0  CPFraction=off  CPFractionValue=0.55  removeDCSubcarriers=off  enableResetInputPort=off  Normalize=off  RoundingMethod=Floor  SimulateUsing=Code generation
  ctrl_gen : Subsystem
  data_out : Outport  OutDataTypeStr=fixdt(1,16,12)
  ctrl_out : Outport  Port=2  OutDataTypeStr=Bus: samplecontrol
  wires:
  ofdm_sym/1 -> OFDM Demodulator/1
  valid_in/1 -> OFDM Demodulator/2
  OFDM Demodulator/1 -> ctrl_gen/1(data_in)
  ctrl_gen/1(data_out) -> data_out/1
  OFDM Demodulator/2 -> ctrl_gen/2(valid_in)
  ctrl_gen/2(ctrl_out) -> ctrl_out/1

== system rx2/process12/OFDM_DEMOD1/OFDM_demod6 ==
  ofdm_sym : Inport
  valid_in : Inport  Port=2  OutDataTypeStr=boolean
  OFDM Demodulator : whdlmod/OFDM Demodulator  OFDMParamsSource=Property  MaxFFTLength=64  FFTLength=1024  CPLength=72  NumLGsC=0  NumRGsC=0  CPFraction=off  CPFractionValue=0.55  removeDCSubcarriers=off  enableResetInputPort=off  Normalize=off  RoundingMethod=Floor  SimulateUsing=Code generation
  ctrl_gen : Subsystem
  data_out : Outport  OutDataTypeStr=fixdt(1,16,12)
  ctrl_out : Outport  Port=2  OutDataTypeStr=Bus: samplecontrol
  wires:
  ofdm_sym/1 -> OFDM Demodulator/1
  valid_in/1 -> OFDM Demodulator/2
  OFDM Demodulator/1 -> ctrl_gen/1(data_in)
  ctrl_gen/1(data_out) -> data_out/1
  OFDM Demodulator/2 -> ctrl_gen/2(valid_in)
  ctrl_gen/2(ctrl_out) -> ctrl_out/1

== system rx2/process12/OFDM_DEMOD1/OFDM_demod7 ==
  ofdm_sym : Inport
  valid_in : Inport  Port=2  OutDataTypeStr=boolean
  OFDM Demodulator : whdlmod/OFDM Demodulator  OFDMParamsSource=Property  MaxFFTLength=64  FFTLength=1024  CPLength=72  NumLGsC=0  NumRGsC=0  CPFraction=off  CPFractionValue=0.55  removeDCSubcarriers=off  enableResetInputPort=off  Normalize=off  RoundingMethod=Floor  SimulateUsing=Code generation
  ctrl_gen : Subsystem
  data_out : Outport  OutDataTypeStr=fixdt(1,16,12)
  ctrl_out : Outport  Port=2  OutDataTypeStr=Bus: samplecontrol
  wires:
  ofdm_sym/1 -> OFDM Demodulator/1
  valid_in/1 -> OFDM Demodulator/2
  OFDM Demodulator/1 -> ctrl_gen/1(data_in)
  ctrl_gen/1(data_out) -> data_out/1
  OFDM Demodulator/2 -> ctrl_gen/2(valid_in)
  ctrl_gen/2(ctrl_out) -> ctrl_out/1

== system rx2/process12/OFDM_DEMOD1/OFDM_demod8 ==
  ofdm_sym : Inport
  valid_in : Inport  Port=2  OutDataTypeStr=boolean
  OFDM Demodulator : whdlmod/OFDM Demodulator  OFDMParamsSource=Property  MaxFFTLength=64  FFTLength=1024  CPLength=72  NumLGsC=0  NumRGsC=0  CPFraction=off  CPFractionValue=0.55  removeDCSubcarriers=off  enableResetInputPort=off  Normalize=off  RoundingMethod=Floor  SimulateUsing=Code generation
  ctrl_gen : Subsystem
  data_out : Outport  OutDataTypeStr=fixdt(1,16,12)
  ctrl_out : Outport  Port=2  OutDataTypeStr=Bus: samplecontrol
  wires:
  ofdm_sym/1 -> OFDM Demodulator/1
  valid_in/1 -> OFDM Demodulator/2
  OFDM Demodulator/1 -> ctrl_gen/1(data_in)
  ctrl_gen/1(data_out) -> data_out/1
  OFDM Demodulator/2 -> ctrl_gen/2(valid_in)
  ctrl_gen/2(ctrl_out) -> ctrl_out/1

== system rx2/process12/decoder/MRC ==
  chan_est_tt : Inport  OutDataTypeStr=fixdt(1,16,12)
  rxSig_tt : Inport  Port=2  OutDataTypeStr=fixdt(1,16,12)
  valid_tt : Inport  Port=3  OutDataTypeStr=boolean
  Add : Sum  Inputs=++++++++
  Add1 : Sum  Inputs=++++++++  OutDataTypeStr=fixdt(1,16,10)  SaturateOnIntegerOverflow=on
  Add2 : Sum  Inputs=++++++++  AccumDataTypeStr=fixdt(1,35,24)
  Constant : Constant  Value=0
  Constant1 : Constant  Value=0
  Demux : Demux  Outputs=8
  Demux1 : Demux  Outputs=8
  Detect Rise Positive1 : hdlsllib/Logic and Bit Operations/Detect Rise Positive  vinit=0  OutDataTypeStr=boolean
  Math Reciprocal : Math  Operator=reciprocal  SignedPower=on  OutDataTypeStr=fixdt(1,19,12)
  Math Reciprocal1 : Math  Operator=reciprocal  SignedPower=on
  Product : Product  OutDataTypeStr=fixdt(1,16,12)
  Product{1..8} (8 alike) : Product  OutDataTypeStr=fixdt(1,33,24)
  Product9 : Product  OutDataTypeStr=fixdt(1,16,9)
  Sqrt{1..8} (8 alike) : Sqrt  OutDataTypeStr=fixdt(1,16,12)  IntermediateResultsDataTypeStr=Inherit: Inherit from input
  Square{,1..7} (8 alike) : Math  Operator=magnitude^2  SignedPower=on  OutDataTypeStr=fixdt(1,32,24)  RndMeth=Zero
  Switch1 : Switch  Criteria=u2 ~= 0  SaturateOnIntegerOverflow=off  InputSameDT=off
  Switch2 : Switch  Criteria=u2 ~= 0  SaturateOnIntegerOverflow=off  InputSameDT=off
  Transpose{,1..7} (8 alike) : Math  Operator=hermitian  SignedPower=on  RndMeth=Zero
  G_k_1 : Outport
  r_k : Outport  Port=2
  start : Outport  Port=3  OutDataTypeStr=boolean  VectorParamsAs1DForOutWhenUnconnected=off
  valid : Outport  Port=4  OutDataTypeStr=boolean  VectorParamsAs1DForOutWhenUnconnected=off
  wires:
  Detect Rise Positive1/1 -> start/1
  Switch2/1 -> Product/1
  Constant1/1 -> Switch2/3
  Math Reciprocal/1 -> Switch2/1
  Constant/1 -> Switch1/3
  Switch1/1 -> Product9/1
  Math Reciprocal1/1 -> Switch1/1
  Product/1 -> G_k_1/1  "G_k_1"
  Demux1/2 -> Product2/2
  Square6/1 -> Add/7, Sqrt7/1
  Demux1/5 -> Product5/2
  Sqrt2/1 -> Add1/2
  Demux/5 -> Transpose4/1, Square4/1
  Sqrt5/1 -> Add1/5
  Product6/1 -> Add2/6
  Demux/1 -> Square/1, Transpose/1
  Sqrt1/1 -> Add1/1
  Product5/1 -> Add2/5
  Demux/3 -> Transpose2/1, Square2/1
  Transpose1/1 -> Product2/1
  Sqrt7/1 -> Add1/7
  Transpose2/1 -> Product3/1
  Demux1/3 -> Product3/2
  Square/1 -> Add/1, Sqrt1/1
  Demux1/1 -> Product1/2
  Transpose6/1 -> Product7/1
  Product9/1 -> r_k/1  "r_k"
  Product1/1 -> Add2/1
  Demux/6 -> Transpose5/1, Square5/1
  Add1/1 -> Math Reciprocal/1
  Product7/1 -> Add2/7
  Transpose5/1 -> Product6/1
  Transpose3/1 -> Product4/1
  Square3/1 -> Add/4, Sqrt4/1
  Sqrt3/1 -> Add1/3
  Product2/1 -> Add2/2
  valid_tt/1 -> valid/1, Switch2/2, Switch1/2, Detect Rise Positive1/1
  Square1/1 -> Add/2, Sqrt2/1
  Transpose4/1 -> Product5/1
  Product4/1 -> Add2/4
  Add/1 -> Product/2, Math Reciprocal1/1  "G_k"
  Demux/4 -> Transpose3/1, Square3/1
  rxSig_tt/1 -> Demux1/1
  Transpose/1 -> Product1/1
  Product3/1 -> Add2/3
  Transpose7/1 -> Product8/1
  Add2/1 -> Product9/2
  Square5/1 -> Add/6, Sqrt6/1
  Sqrt6/1 -> Add1/6
  chan_est_tt/1 -> Demux/1
  Demux1/6 -> Product6/2
  Demux1/8 -> Product8/2
  Square7/1 -> Add/8, Sqrt8/1
  Sqrt4/1 -> Add1/4
  Demux/7 -> Transpose6/1, Square6/1
  Sqrt8/1 -> Add1/8
  Demux1/4 -> Product4/2
  Product8/1 -> Add2/8
  Square4/1 -> Add/5, Sqrt5/1
  Square2/1 -> Add/3, Sqrt3/1
  Demux/2 -> Transpose1/1, Square1/1
  Demux1/7 -> Product7/2
  Demux/8 -> Transpose7/1, Square7/1

== system rx2/process12/decoder/deinterleave ==
  data_tt : Inport  SampleTime=1
  valid_tt : Inport  Port=2  OutDataTypeStr=boolean  SampleTime=1
  Compare To Constant : simulink/Logic and Bit Operations/Compare To Constant  relop=>  const=length/2-1  OutDataTypeStr=boolean
  Data Type Conversion : DataTypeConversion  OutDataTypeStr=boolean  SaturateOnIntegerOverflow=off  RndMeth=Floor
  Delay : Delay  DelayLength=1  InitialCondition=0
  Delay1 : Delay  DelayLength=1  InitialCondition=0
  Delay2 : Delay  DelayLength=1  InitialCondition=0
  Detect Fall Nonpositive : simulink/Logic and Bit Operations/Detect Fall Nonpositive  vinit=0  OutDataTypeStr=boolean
  Detect Rise Positive : simulink/Logic and Bit Operations/Detect Rise Positive  vinit=0  OutDataTypeStr=boolean
  HDL Counter : hdlsllib/Sources/HDL Counter  CountType=Count limited  CountInit=0  CountStep=1  CountMax=1  CountFromType=Initial value  CountFrom=0  CountResetPort=on  CountLoadPort=off  CountEnbPort=on  CountDirPort=off  CountHitOutputPort=off  CountDataType=Unsigned  CountWordLen=8  CountFracLen=0  CountSampTime=1
  HDL Counter1 : hdlsllib/Sources/HDL Counter  CountType=Count limited  CountInit=0  CountStep=1  CountMax=length-1  CountFromType=Initial value  CountFrom=0  CountResetPort=on  CountLoadPort=off  CountEnbPort=on  CountDirPort=off  CountHitOutputPort=off  CountDataType=Unsigned  CountWordLen=32  CountFracLen=0  CountSampTime=1
  HDL FIFO : hdlsllib/HDL RAMs/HDL FIFO  fifo_size=length/2  mode=Classic  ratio=1  push_msg=Ignore  pop_msg=Ignore  show_empty=off  show_full=off  show_num=off  LabelModeActiveChoice_Mode=Classic  rst_port=off
  HDL FIFO1 : hdlsllib/HDL RAMs/HDL FIFO  fifo_size=length/2  mode=Classic  ratio=1  push_msg=Ignore  pop_msg=Ignore  show_empty=off  show_full=off  show_num=off  LabelModeActiveChoice_Mode=Classic  rst_port=off
  Logical Operator : Logic  Operator=NOT  AllPortsSameDT=off  OutDataTypeStr=boolean
  Logical Operator1 : Logic  Operator=XOR  AllPortsSameDT=off  OutDataTypeStr=boolean
  Logical Operator2 : Logic  AllPortsSameDT=off  OutDataTypeStr=boolean
  Subsystem : Subsystem  mask{valid_length=length/2}
      mask prompts: valid_length "The length of valid"
      mask DialogControl Control2 Prompt: Latency=2
  Subsystem1 : Subsystem  mask{valid_length=length}
      mask prompts: valid_length "The length of valid"
      mask DialogControl Control2 Prompt: Latency=2
  Switch : Switch  Criteria=u2 > Threshold  SaturateOnIntegerOverflow=off  InputSameDT=off
  data_out : Outport
  valid_out : Outport  Port=2
  wires:
  Switch/1 -> data_out/1
  Subsystem1/1(valid_out) -> valid_out/1
  HDL FIFO/1 -> Switch/1
  Data Type Conversion/1 -> Logical Operator1/1, HDL FIFO1/2  "valid0"
  HDL Counter/1 -> Data Type Conversion/1
  Logical Operator1/1 -> HDL FIFO/2  "valid1"
  data_tt/1 -> HDL FIFO/1, HDL FIFO1/1
  HDL Counter1/1 -> Compare To Constant/1
  Detect Rise Positive/1 -> Subsystem1/1(start)
  Compare To Constant/1 -> Detect Fall Nonpositive/1, Delay/1
  Detect Fall Nonpositive/1 -> Logical Operator2/2
  Delay1/1 -> HDL FIFO/3, Delay2/1
  valid_tt/1 -> HDL Counter/2, Logical Operator/1, Logical Operator1/2, HDL Counter1/2
  Delay2/1 -> Switch/2
  HDL FIFO1/1 -> Switch/3
  Logical Operator/1 -> HDL Counter/1, HDL Counter1/1
  Subsystem/1(valid_out) -> HDL FIFO1/3
  Delay/1 -> Logical Operator2/1, Detect Rise Positive/1, Delay1/1
  Logical Operator2/1 -> Subsystem/1(start)

== system rx2/process12/decoder/p-p ==
  data_in : Inport  OutDataTypeStr=boolean  PortDimensions=64
  start_in : Inport  Port=2  OutDataTypeStr=boolean  PortDimensions=1
  valid : Inport  Port=3  OutDataTypeStr=boolean  PortDimensions=1
  Compare To Constant : hdlsllib/Logic and Bit Operations/Compare To Constant  relop===  const=64  OutDataTypeStr=boolean
  Compare To Constant1 : hdlsllib/Logic and Bit Operations/Compare To Constant  relop=<=  const=72  OutDataTypeStr=boolean
  Compare To Constant2 : hdlsllib/Logic and Bit Operations/Compare To Constant  relop===  const=1  OutDataTypeStr=boolean
  Compare To Constant3 : hdlsllib/Logic and Bit Operations/Compare To Constant  relop===  const=528  OutDataTypeStr=boolean
  Compare To Constant4 : hdlsllib/Logic and Bit Operations/Compare To Constant  relop=<=  const=528  OutDataTypeStr=boolean
  Delay : Delay  DelayLength=1  InitialCondition=0
  Delay1 : Delay  DelayLength=1  InitialCondition=0
  Ground : Ground
  HDL Counter : hdlsllib/Sources/HDL Counter  CountType=Count limited  CountInit=0  CountStep=1  CountMax=2000  CountFromType=Specify  CountFrom=0  CountResetPort=on  CountLoadPort=off  CountEnbPort=on  CountDirPort=off  CountHitOutputPort=off  CountDataType=Unsigned  CountWordLen=16  CountFracLen=0  CountSampTime=1
  HDL Counter1 : hdlsllib/Sources/HDL Counter  CountType=Count limited  CountInit=1  CountStep=1  CountMax=64  CountFromType=Specify  CountFrom=1  CountResetPort=on  CountLoadPort=off  CountEnbPort=on  CountDirPort=off  CountHitOutputPort=off  CountDataType=Unsigned  CountWordLen=16  CountFracLen=0  CountSampTime=1
  HDL Counter2 : hdlsllib/Sources/HDL Counter  CountType=Count limited  CountInit=0  CountStep=1  CountMax=100  CountFromType=Specify  CountFrom=0  CountResetPort=on  CountLoadPort=off  CountEnbPort=on  CountDirPort=off  CountHitOutputPort=off  CountDataType=Unsigned  CountWordLen=16  CountFracLen=0  CountSampTime=1
  HDL Counter3 : hdlsllib/Sources/HDL Counter  CountType=Count limited  CountInit=1  CountStep=1  CountMax=64*2  CountFromType=Initial value  CountFrom=1  CountResetPort=on  CountLoadPort=off  CountEnbPort=on  CountDirPort=off  CountHitOutputPort=off  CountDataType=Unsigned  CountWordLen=8  CountFracLen=0  CountSampTime=1
  HDL Counter4 : hdlsllib/Sources/HDL Counter  CountType=Count limited  CountInit=0  CountStep=1  CountMax=1000  CountFromType=Initial value  CountFrom=0  CountResetPort=on  CountLoadPort=off  CountEnbPort=on  CountDirPort=off  CountHitOutputPort=off  CountDataType=Unsigned  CountWordLen=16  CountFracLen=0  CountSampTime=1
  HDL Counter5 : hdlsllib/Sources/HDL Counter  CountType=Count limited  CountInit=1  CountStep=1  CountMax=1000  CountFromType=Initial value  CountFrom=1  CountResetPort=on  CountLoadPort=off  CountEnbPort=on  CountDirPort=off  CountHitOutputPort=off  CountDataType=Unsigned  CountWordLen=16  CountFracLen=0  CountSampTime=1
  Logical Operator1 : Logic  Operator=NOT  AllPortsSameDT=off  OutDataTypeStr=boolean
  Logical Operator2 : Logic  Operator=NOT  AllPortsSameDT=off  OutDataTypeStr=boolean
  Logical Operator3 : Logic  AllPortsSameDT=off  OutDataTypeStr=boolean
  Logical Operator5 : Logic  Operator=NOT  AllPortsSameDT=off  OutDataTypeStr=boolean
  Logical Operator6 : Logic  AllPortsSameDT=off  OutDataTypeStr=boolean
  Sample Control Bus Creator : whdlutilities/Sample Control Bus Creator
  Subsystem : Subsystem  mask{valid_length=20*64}
      mask prompts: valid_length "The length of valid"
      mask DialogControl Control2 Prompt: Latency=2
  Subsystem2 : Subsystem  mask{data_type=boolean, address_len=16}
      mask prompts: data_type "the type of input data"; address_len "the length of address"
      mask DialogControl ParameterGroupVar Prompt: 参数
  Switch : Switch  Criteria=u2 ~= 0  SaturateOnIntegerOverflow=off  InputSameDT=off
  p_s_new : Subsystem
  data : Outport
  ctrl : Outport  Port=2
  wires:
  HDL Counter4/1 -> Compare To Constant3/1, Compare To Constant2/1
  Logical Operator1/1 -> HDL Counter2/1, HDL Counter1/1
  Logical Operator3/1 -> HDL Counter5/2, Logical Operator6/2
  valid/1 -> HDL Counter/2, Subsystem2/3(wr_en1), Logical Operator5/1
  HDL Counter/1 -> Subsystem2/2(wr_addr)
  start_in/1 -> Subsystem/1(start)
  Compare To Constant/1 -> HDL Counter2/2
  Logical Operator2/1 -> HDL Counter5/1, HDL Counter3/1
  Logical Operator5/1 -> HDL Counter/1
  data_in/1 -> Subsystem2/1(data1)
  HDL Counter2/1 -> Subsystem2/4(rd_addr)
  HDL Counter3/1 -> Compare To Constant1/1
  Compare To Constant1/1 -> Logical Operator3/2
  HDL Counter1/1 -> Compare To Constant/1
  Compare To Constant2/1 -> Sample Control Bus Creator/1
  Compare To Constant3/1 -> Sample Control Bus Creator/2, HDL Counter4/1
  Delay/1 -> Switch/2, Sample Control Bus Creator/3
  Delay1/1 -> Switch/1
  Sample Control Bus Creator/1 -> ctrl/1
  HDL Counter5/1 -> Compare To Constant4/1
  Compare To Constant4/1 -> Logical Operator6/1
  Logical Operator6/1 -> Delay/1, HDL Counter4/2
  Subsystem/1(valid_out) -> p_s_new/2(valid), Logical Operator3/1, Logical Operator2/1, HDL Counter3/2, Logical Operator1/1, HDL Counter1/2
  Subsystem2/1(rd_dout) -> p_s_new/1(data_in)
  p_s_new/1(data_out) -> Delay1/1
  Subsystem/3(end_out) -> p_s_new/3(end)
  Switch/1 -> data/1
  Ground/1 -> Switch/3

== system rx2/process12/decoder/rate recover ==
  demod : Inport
  valid_in : Inport  Port=2
  start_in : Inport  Port=3
  Compare To Constant : hdlsllib/Logic and Bit Operations/Compare To Constant  relop=<=  const=384  OutDataTypeStr=boolean
  Compare To Constant1 : hdlsllib/Logic and Bit Operations/Compare To Constant  relop=>=  const=577  OutDataTypeStr=boolean
  Compare To Constant2 : hdlsllib/Logic and Bit Operations/Compare To Constant  relop=<=  const=1776  OutDataTypeStr=boolean
  Compare To Constant3 : hdlsllib/Logic and Bit Operations/Compare To Constant  relop=>=  const=385  OutDataTypeStr=boolean
  Compare To Constant4 : hdlsllib/Logic and Bit Operations/Compare To Constant  relop=<=  const=576  OutDataTypeStr=boolean
  Compare To Constant5 : hdlsllib/Logic and Bit Operations/Compare To Constant  relop=>=  const=1777  OutDataTypeStr=boolean
  Compare To Constant6 : hdlsllib/Logic and Bit Operations/Compare To Constant  relop=<=  const=3600  OutDataTypeStr=boolean
  Constant : Constant  Value=0
  Constant1 : Constant  Value=0
  Delay{,1..4} (5 alike) : Delay  InitialCondition=0
  HDL Counter : hdlsllib/Sources/HDL Counter  CountType=Count limited  CountInit=1  CountStep=1  CountMax=10000  CountFromType=Initial value  CountFrom=1  CountResetPort=on  CountLoadPort=off  CountEnbPort=on  CountDirPort=off  CountHitOutputPort=off  CountDataType=Unsigned  CountWordLen=16  CountFracLen=0  CountSampTime=1
  HDL Counter1 : hdlsllib/Sources/HDL Counter  CountType=Count limited  CountInit=0  CountStep=1  CountMax=10000  CountFromType=Initial value  CountFrom=0  CountResetPort=on  CountLoadPort=off  CountEnbPort=on  CountDirPort=off  CountHitOutputPort=off  CountDataType=Unsigned  CountWordLen=16  CountFracLen=0  CountSampTime=1
  HDL Counter3 : hdlsllib/Sources/HDL Counter  CountType=Count limited  CountInit=1  CountStep=1  CountMax=10000  CountFromType=Initial value  CountFrom=1  CountResetPort=on  CountLoadPort=off  CountEnbPort=on  CountDirPort=off  CountHitOutputPort=off  CountDataType=Unsigned  CountWordLen=16  CountFracLen=0  CountSampTime=1
  Logical Operator : Logic  Operator=NOT  AllPortsSameDT=off  OutDataTypeStr=boolean
  Logical Operator{1,3..4,6..7} (5 alike) : Logic  AllPortsSameDT=off  OutDataTypeStr=boolean
  Logical Operator5 : Logic  Operator=OR  AllPortsSameDT=off  OutDataTypeStr=boolean
  Logical Operator8 : Logic  Operator=NOT  AllPortsSameDT=off  OutDataTypeStr=boolean
  Simple Dual Port RAM : hdlsllib/HDL RAMs/Simple Dual Port RAM  ram_size=16
  Subsystem : Subsystem  mask{valid_length=3600}
      mask prompts: valid_length "The length of valid"
      mask DialogControl Control2 Prompt: Latency=2
  Switch : Switch  Criteria=u2 ~= 0  SaturateOnIntegerOverflow=off  InputSameDT=off
  Switch1 : Switch  Criteria=u2 ~= 0  OutDataTypeStr=fixdt(1,16,9)  SaturateOnIntegerOverflow=off  InputSameDT=off
  rate_recover : Outport  PortDimensions=1
  start_out : Outport  Port=2  OutDataTypeStr=boolean
  end_out : Outport  Port=3  OutDataTypeStr=boolean
  valid_out : Outport  Port=4  OutDataTypeStr=boolean
  wires:
  HDL Counter1/1 -> Simple Dual Port RAM/4  "rd_addr"
  Logical Operator6/1 -> HDL Counter1/2  "1"
  Delay4/1 -> Switch1/2  "3"
  Delay3/1 -> Switch/2  "2"
  HDL Counter3/1 -> Compare To Constant2/1, Compare To Constant3/1, Compare To Constant4/1, Compare To Constant5/1, Compare To Constant6/1, Compare To Constant/1, Compare To Constant1/1  "count"
  Logical Operator8/1 -> HDL Counter3/1, HDL Counter1/1
  Delay/1 -> valid_out/1, Logical Operator7/2  "valid_out"
  demod/1 -> Simple Dual Port RAM/1
  Delay2/1 -> end_out/1  "end_out"
  Compare To Constant/1 -> Logical Operator5/1
  Logical Operator5/1 -> Logical Operator6/1
  Switch1/1 -> rate_recover/1  "data_out"
  Switch/1 -> Switch1/3  "2_out"
  Constant/1 -> Switch/1
  Logical Operator4/1 -> Logical Operator7/1
  Compare To Constant4/1 -> Logical Operator3/2
  start_in/1 -> Subsystem/1(start)
  Simple Dual Port RAM/1 -> Switch/3  "rd_dout"
  Logical Operator7/1 -> Delay4/1  "3"
  Delay1/1 -> start_out/1  "start_out"
  valid_in/1 -> Logical Operator/1, HDL Counter/2, Simple Dual Port RAM/3
  Compare To Constant2/1 -> Logical Operator1/2
  Compare To Constant1/1 -> Logical Operator1/1
  Compare To Constant6/1 -> Logical Operator4/2
  HDL Counter/1 -> Simple Dual Port RAM/2  "wr_addr"
  Subsystem/3(end_out) -> Delay2/1  "end"
  Compare To Constant3/1 -> Logical Operator3/1
  Logical Operator1/1 -> Logical Operator5/2
  Logical Operator/1 -> HDL Counter/1
  Subsystem/2(start_out) -> Delay1/1  "start"
  Constant1/1 -> Switch1/1
  Subsystem/1(valid_out) -> HDL Counter3/2, Delay/1, Logical Operator6/2, Logical Operator8/1
  Logical Operator3/1 -> Delay3/1
  Compare To Constant5/1 -> Logical Operator4/1
